simulink subsystem "Controller"  (R2024a)
settings: Solver=VariableStepAuto  StartTime=0.0  StopTime=10.0  RelTol=1e-3
undefined symbols (not defined in the file): A, MPC, N, physics, PWM
libraries: mpclib x3, robotlib x3, simulink x2, ros2lib x2, sharedTrackingLibrary x1
settings Model: Creator=Lamarre  LastModifiedBy=nimai
settings SolverCC: AlgebraicLoopSolver=TrustRegion
settings DebuggingCC: UnconnectedInputMsg=warning  UnconnectedOutputMsg=warning  UnconnectedLineMsg=warning
settings ModelReferenceCC: EnableRefExpFcnMdlSchedulingChecks=on
settings RTWCC: GPUComputeCapability=3.5  DLArmComputeVersion=19.05

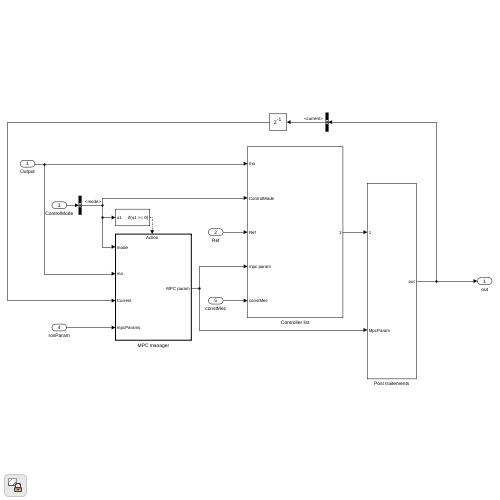
[thumbnail: Simulink's stored preview of the top-level diagram]
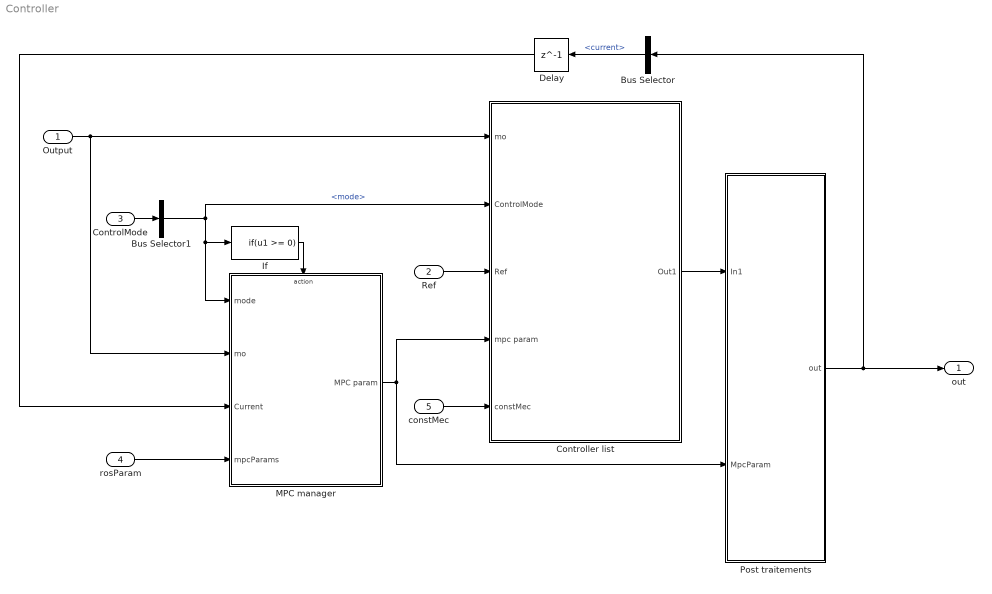
== system Controller ==
  Output : Inport
  Ref : Inport  Port=2
  ControlMode : Inport  Port=3
  rosParam : Inport  Port=4
  constMec : Inport  Port=5
  Bus Selector : BusSelector  OutputSignals=current
  Bus Selector1 : BusSelector  OutputSignals=mode
  Controller list : Subsystem
  Delay : Delay  DelayLength=1  InitialCondition=zeros(1,8)  SampleTime=MPC.Ts
  If : If  IfExpression=u1 >= 0  ShowElse=off
  MPC manager : Subsystem
  Post traitements : Subsystem
  out : Outport
  wires:
  Output/1 -> MPC manager/2(mo), Controller list/1(mo)
  ControlMode/1 -> Bus Selector1/1
  Ref/1 -> Controller list/3(Ref)
  Controller list/1(Out1) -> Post traitements/1(In1)
  Post traitements/1(out) -> out/1, Bus Selector/1
  Delay/1 -> MPC manager/3(Current)
  MPC manager/1(MPC param) -> Post traitements/2(MpcParam), Controller list/4(mpc param)
  Bus Selector/1 -> Delay/1  "<current>"
  Bus Selector1/1 -> Controller list/2(ControlMode), If/1, MPC manager/1(mode)  "<mode>"
  If/1 -> MPC manager/Action
  rosParam/1 -> MPC manager/4(mpcParams)
  constMec/1 -> Controller list/5(constMec)

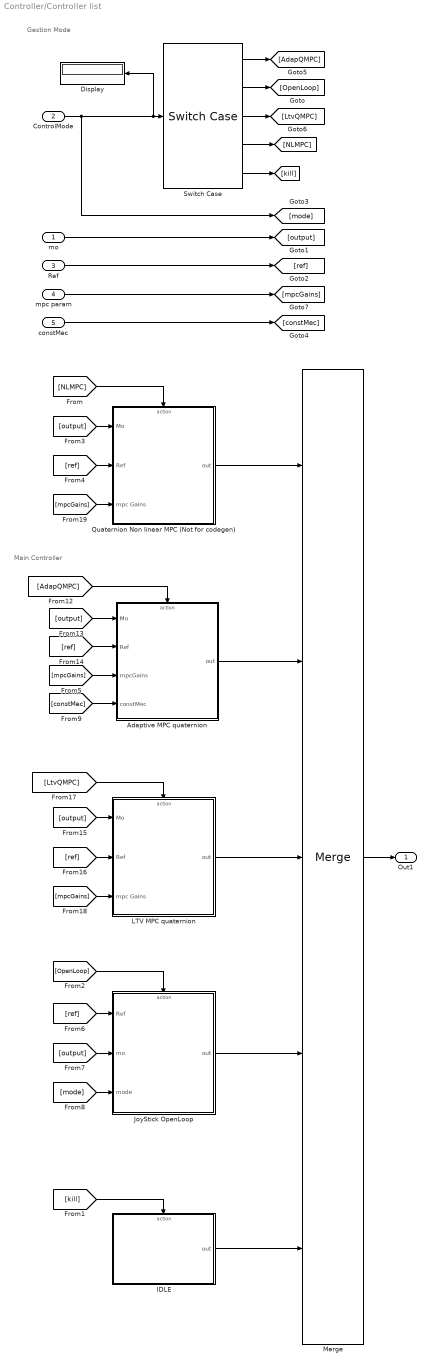
== system Controller/Controller list ==
  note: Gestion Mode
  note: Main Controller
  mo : Inport
  ControlMode : Inport  Port=2
  Ref : Inport  Port=3
  mpc param : Inport  Port=4
  constMec : Inport  Port=5
  "Adaptive MPC quaternion " : Subsystem
  Display : Display
  IDLE : Subsystem  TreatAsAtomicUnit=on
  JoyStick OpenLoop : Subsystem  TreatAsAtomicUnit=on
  "LTV MPC quaternion " : Subsystem
  Merge : Merge  Inputs=5
  Quaternion Non linear MPC (Not for codegen) : Subsystem
  Switch Case : SwitchCase  CaseConditions="{ mode.control.adapQMpcMode,  mode.control.openLoopMode,    mode.control.LtvQMpcMode, mode.control.NlmpcMode}"
  Out1 : Outport
  wires:
  [constMec] -> "Adaptive MPC quaternion "/4(constMec)
  constMec/1 -> [constMec]
  JoyStick OpenLoop/1(out) -> Merge/4
  "LTV MPC quaternion "/1(out) -> Merge/3
  "Adaptive MPC quaternion "/1(out) -> Merge/2
  Switch Case/4 -> [NLMPC]
  Switch Case/3 -> [LtvQMPC]
  Switch Case/1 -> [AdapQMPC]
  [mpcGains] -> Quaternion Non linear MPC (Not for codegen)/3(mpc Gains)
  [mpcGains] -> "LTV MPC quaternion "/3(mpc Gains)
  [mpcGains] -> "Adaptive MPC quaternion "/3(mpcGains)
  mpc param/1 -> [mpcGains]
  Switch Case/2 -> [OpenLoop]
  Ref/1 -> [ref]
  mo/1 -> [output]
  ControlMode/1 -> [mode], Switch Case/1, Display/1
  Switch Case/5 -> [kill]
  [output] -> Quaternion Non linear MPC (Not for codegen)/1(Mo)
  [AdapQMPC] -> "Adaptive MPC quaternion "/Action
  [ref] -> "Adaptive MPC quaternion "/2(Ref)
  [kill] -> IDLE/Action
  [output] -> "LTV MPC quaternion "/1(Mo)
  [ref] -> Quaternion Non linear MPC (Not for codegen)/2(Ref)
  Merge/1 -> Out1/1
  [output] -> JoyStick OpenLoop/2(mo)
  Quaternion Non linear MPC (Not for codegen)/1(out) -> Merge/1
  [ref] -> "LTV MPC quaternion "/2(Ref)
  [output] -> "Adaptive MPC quaternion "/1(Mo)
  [LtvQMPC] -> "LTV MPC quaternion "/Action
  IDLE/1(out) -> Merge/5
  [NLMPC] -> Quaternion Non linear MPC (Not for codegen)/Action
  [mode] -> JoyStick OpenLoop/3(mode)
  [ref] -> JoyStick OpenLoop/1(Ref)
  [OpenLoop] -> JoyStick OpenLoop/Action

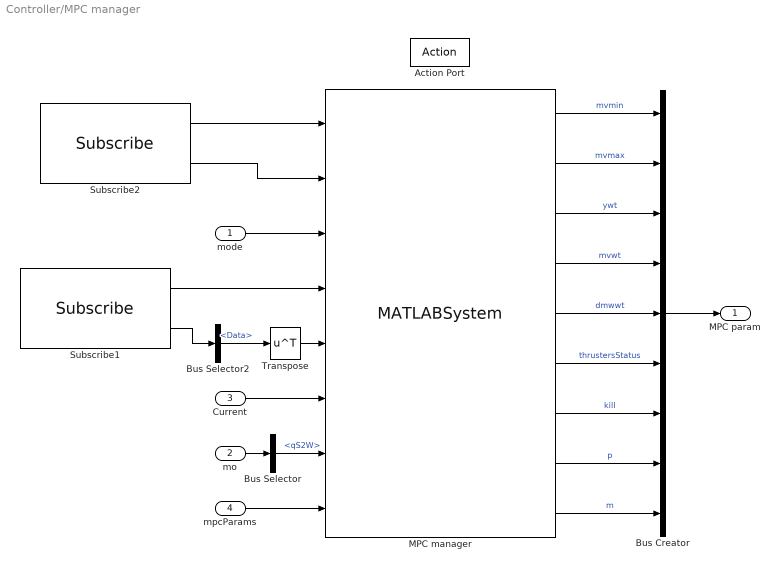
== system Controller/MPC manager ==
  mode : Inport
  mo : Inport  Port=2
  Current : Inport  Port=3
  mpcParams : Inport  Port=4
  Action Port : ActionPort  InitializeStates=reset
  Bus Creator : BusCreator  Inputs=9
  Bus Selector : BusSelector  OutputSignals=qS2W
  Bus Selector2 : BusSelector  OutputSignals=Data
  MPC manager : MATLABSystem  System=mpcManager  mpcConst=MPC  mode=mode  SimulateUsing=Code generation
      mask Type: mpcManager
      mask Display:
      | disp('mpcManager');
      | port_label('input',1,'newRosGains');
      | port_label('input',2,'rosGains');
      | port_label('input',3,'mode');
      | port_label('input',4,'newReadCurrent');
      | port_label('input',5,'readCurrent');
      | port_label('input',6,'estimatedCurrent');
      | port_label('input',7,'mo');
      | port_label('input',8,'mpcParams');
      | port_label('output',1,'mvmin');
      | port_label('output',2,'mvmax');
      | port_label('output',3,'ywt');
      | port_label('output',4,'mvwt');
      | port_label('output',5,'dmwwt');
      | port_label('output',6,'tInfo');
      | port_label('output',7,'kill');
      | port_label('output',8,'p');
      | port_label('output',9,'m');
  Subscribe1 : ros2lib/Subscribe  topicSource=Specify your own  topic=/provider_power/current_not  messageType=std_msgs/Float64MultiArray  sampleTime=-1  QOSHistory=Keep last  QOSDepth=1  QOSReliability=Reliable  QOSDurability=Volatile  QOSDeadline=Inf  QOSLifespan=Inf  QOSLiveliness=Automatic  QOSLeaseDuration=Inf  QOSAvoidROSNamespaceConventions=off
  Subscribe2 : ros2lib/Subscribe  topicSource=Specify your own  topic=/proc_control/set_mpc_gains  messageType=sonia_common_ros2/MpcGains  sampleTime=-1  QOSHistory=Keep last  QOSDepth=1  QOSReliability=Reliable  QOSDurability=Volatile  QOSDeadline=Inf  QOSLifespan=Inf  QOSLiveliness=Automatic  QOSLeaseDuration=Inf  QOSAvoidROSNamespaceConventions=off
  Transpose : Math  Operator=transpose
  MPC param : Outport
  wires:
  mpcParams/1 -> MPC manager/8
  MPC manager/9 -> Bus Creator/9  "m"
  MPC manager/8 -> Bus Creator/8  "p"
  Bus Selector/1 -> MPC manager/7  "<qS2W>"
  mo/1 -> Bus Selector/1
  MPC manager/7 -> Bus Creator/7  "kill"
  MPC manager/6 -> Bus Creator/6  "thrustersStatus"
  Subscribe2/2 -> MPC manager/2
  Subscribe2/1 -> MPC manager/1
  mode/1 -> MPC manager/3
  Subscribe1/1 -> MPC manager/4
  Transpose/1 -> MPC manager/5
  Current/1 -> MPC manager/6
  Bus Creator/1 -> MPC param/1
  MPC manager/3 -> Bus Creator/3  "ywt"
  MPC manager/5 -> Bus Creator/5  "dmwwt"
  MPC manager/4 -> Bus Creator/4  "mvwt"
  MPC manager/2 -> Bus Creator/2  "mvmax"
  MPC manager/1 -> Bus Creator/1  "mvmin"
  Bus Selector2/1 -> Transpose/1  "<Data>"
  Subscribe1/2 -> Bus Selector2/1

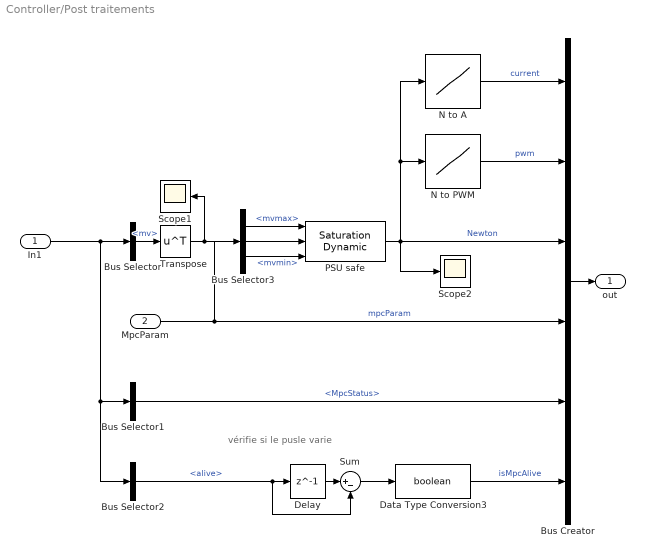
== system Controller/Post traitements ==
  note: vérifie si le pusle varie
  In1 : Inport
  MpcParam : Inport  Port=2
  Bus Creator : BusCreator  Inputs=6
  Bus Selector : BusSelector  OutputSignals=mv
  Bus Selector1 : BusSelector  OutputSignals=MpcStatus
  Bus Selector2 : BusSelector  OutputSignals=alive
  Bus Selector3 : BusSelector  OutputSignals=mvmax,mvmin
  Data Type Conversion3 : DataTypeConversion  OutDataTypeStr=boolean  RndMeth=Nearest  SaturateOnIntegerOverflow=off
  Delay : Delay  DelayLength=1  SampleTime=MPC.Ts
  N to A : Lookup_n-D  NumberOfTableDimensions=1  BreakpointsForDimension1=N  BeginIndexSearchUsingPreviousIndexResult=on  Table=A  InterpMethod=Nearest  ExtrapMethod=Clip  DiagnosticForOutOfRangeInput=Warning  RemoveProtectionInput=on  InternalRulePriority=Speed  OutDataTypeStr=uint16  RndMeth=Simplest
  N to PWM : Lookup_n-D  NumberOfTableDimensions=1  BreakpointsForDimension1=N  BeginIndexSearchUsingPreviousIndexResult=on  Table=PWM  InterpMethod=Nearest  ExtrapMethod=Clip  DiagnosticForOutOfRangeInput=Warning  RemoveProtectionInput=on  InternalRulePriority=Speed  OutDataTypeStr=uint16  RndMeth=Simplest
  PSU safe : simulink/Discontinuities/Saturation Dynamic  OutMin=[]  OutMax=[]  OutDataTypeStr=Inherit: Same as second input  OutDataType=fixdt(1, 16)  OutScaling=2^-10  DoSatur=off
  Scope1 : Scope
  Scope2 : Scope
  Sum : Sum  Inputs=|+-
  Transpose : Math  Operator=transpose
  out : Outport
  wires:
  Bus Selector3/2 -> PSU safe/3  "<mvmin>"
  Bus Selector3/1 -> PSU safe/1  "<mvmax>"
  Transpose/1 -> PSU safe/2, Scope1/1
  Bus Selector2/1 -> Delay/1, Sum/2  "<alive>"
  Data Type Conversion3/1 -> Bus Creator/6  "isMpcAlive"
  Delay/1 -> Sum/1
  Sum/1 -> Data Type Conversion3/1
  MpcParam/1 -> Bus Selector3/1, Bus Creator/4  "mpcParam"
  Bus Creator/1 -> out/1
  N to A/1 -> Bus Creator/1  "current"
  PSU safe/1 -> N to PWM/1, N to A/1, Bus Creator/3, Scope2/1  "Newton"
  In1/1 -> Bus Selector1/1, Bus Selector2/1, Bus Selector/1
  N to PWM/1 -> Bus Creator/2  "pwm"
  Bus Selector/1 -> Transpose/1  "<mv>"
  Bus Selector1/1 -> Bus Creator/5  "<MpcStatus>"

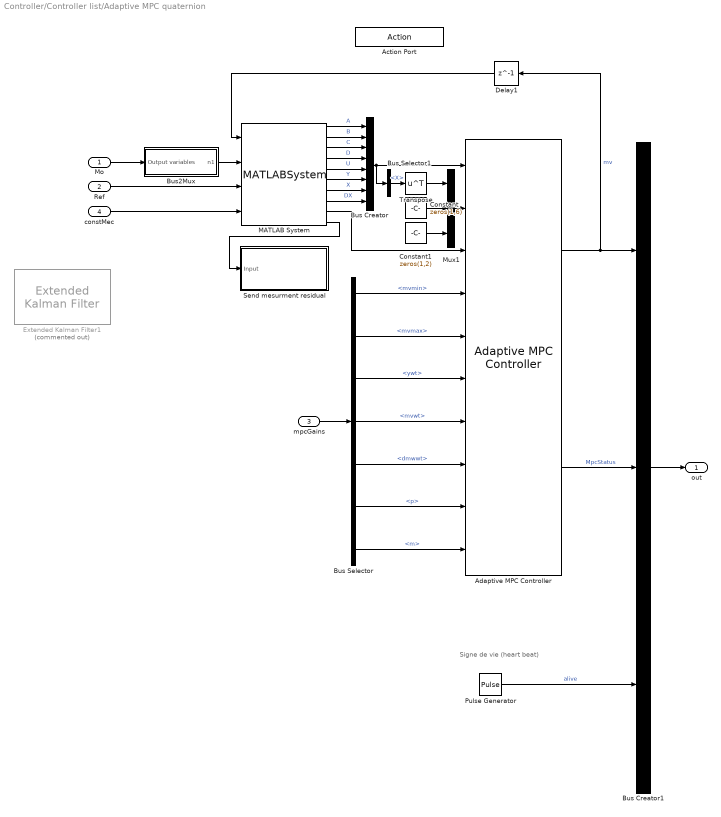
== system Controller/Controller list/Adaptive MPC quaternion  ==
  note: Signe de vie (heart beat)
  Mo : Inport
  Ref : Inport  Port=2
  mpcGains : Inport  Port=3
  constMec : Inport  Port=4
  Action Port : ActionPort  InitializeStates=reset  PropagateVarSize=During execution
  Adaptive MPC Controller : mpclib/Adaptive MPC Controller  SCDEnableBlockLinearizationSpecification=on  mpcobj=Qmpcobj  enable_value=0  updateMPCinCallerWorkspace=on  md_inport=off  mv_inport=off  uref_inport=off  return_cost=off  return_mvseq=off  return_qpstatus=on  return_xseq=off  return_state=off  return_ovseq=off  state_inport=on  isltv_plant=off  umin_inport=on  umax_inport=on  ymin_inport=off  ymax_inport=off  cc_inport=off  ywt_inport=on  uwt_inport=on  duwt_inport=on  rhoeps_inport=off  pm_inport=on  MaximumP=10  HorizonChoice=VariableHorizon  BlockDataType=double  SampleTimeInherited=off  switch_inport=off
  Bus Creator : BusCreator  Inputs=8
  Bus Creator1 : BusCreator  Inputs=3
  Bus Selector : BusSelector  OutputSignals=mvmin,mvmax,ywt,mvwt,dmwwt,p,m
  Bus Selector1 : BusSelector  OutputSignals=X
  Bus2Mux : Subsystem
  Constant : Constant  Value=zeros(1,6)
  Constant1 : Constant  Value=zeros(1,2)
  Delay1 : Delay  DelayLength=1  InitialCondition=zeros(MPC.nu,1)  SampleTime=MPC.Ts
  Extended Kalman Filter1 : sharedTrackingLibrary/Extended Kalman Filter  Commented=on  StateTransitionFcn=QKalmanStateFonction  HasStateTransitionJacobianFcn=off  StateTransitionJacobianFcn=AUVQuatDiscreteJacobianMatrix  HasAdditiveProcessNoise=Additive  ProcessNoise=1  HasTimeVaryingProcessNoise=off  HasStateTransitionFcnExtraArgument=1  InitialState=[0,0,0.31,1,0,0,0,0,0,0,0,0,0,0,0,0,0,0,0,0,0]  InitialStateCovariance=1  MeasurementFcn1=QKalmanMesuredFonction  HasMeasurementJacobianFcn1=off  HasMeasurementEnablePort1=off  HasAdditiveMeasurementNoise1=Additive  MeasurementNoise1=[1,1,1,1,1,1,1,1,1,1,1,1,1]  HasTimeVaryingMeasurementNoise1=off  HasMeasurementFcnExtraArgument1=0  HasMeasurementWrapping1=off  MeasurementFcn2=myMeasurementFcn  HasMeasurementJacobianFcn2=off  HasMeasurementEnablePort2=off  HasAdditiveMeasurementNoise2=Nonadditive  MeasurementNoise2=1  HasTimeVaryingMeasurementNoise2=off  HasMeasurementFcnExtraArgument2=0  HasMeasurementWrapping2=off  MeasurementFcn3=myMeasurementFcn  HasMeasurementJacobianFcn3=off  HasMeasurementEnablePort3=off  HasAdditiveMeasurementNoise3=Additive  MeasurementNoise3=1  HasTimeVaryingMeasurementNoise3=off  HasMeasurementFcnExtraArgument3=0  HasMeasurementWrapping3=off  MeasurementFcn4=myMeasurementFcn  HasMeasurementJacobianFcn4=off  HasMeasurementEnablePort4=off  HasAdditiveMeasurementNoise4=Additive  MeasurementNoise4=1  HasTimeVaryingMeasurementNoise4=off  HasMeasurementFcnExtraArgument4=0  HasMeasurementWrapping4=off  MeasurementFcn5=myMeasurementFcn  HasMeasurementJacobianFcn5=off  HasMeasurementEnablePort5=off  HasAdditiveMeasurementNoise5=Additive  MeasurementNoise5=1  HasTimeVaryingMeasurementNoise5=off  HasMeasurementFcnExtraArgument5=0  HasMeasurementWrapping5=off  EnableMultirate=off  StateTransitionFcnSampleTime=1  MeasurementFcn1SampleTime=1  MeasurementFcn2SampleTime=1  MeasurementFcn3SampleTime=1  MeasurementFcn4SampleTime=1  MeasurementFcn5SampleTime=1  UseCurrentEstimator=on  OutputStateCovariance=off  DataType=double  SampleTime=MPC.Ts  NumberOfMeasurements=1
  MATLAB System : MATLABSystem  System=TrimPlant  MPC=MPC  useDynamicsConst=on  SimulateUsing=Code generation
      mask Type: TrimPlant
      mask Display:
      | disp('TrimPlant');
      | port_label('input',1,'u');
      | port_label('input',2,'y');
      | port_label('input',3,'ref');
      | port_label('input',4,'constMec');
      | port_label('output',1,'A');
      | port_label('output',2,'B');
      | port_label('output',3,'C');
      | port_label('output',4,'D');
      | port_label('output',5,'U');
      | port_label('output',6,'Y');
      | port_label('output',7,'X');
      | port_label('output',8,'DX');
      | port_label('output',9,'ref');
      | port_label('output',10,'Z');
  Mux1 : Mux  Inputs=3
  Pulse Generator : DiscretePulseGenerator  SampleTime=MPC.Ts
  "Send mesurment residual " : Subsystem
  Transpose : Math  Operator=transpose
  out : Outport
  wires:
  MATLAB System/10 -> "Send mesurment residual "/1(Input)
  constMec/1 -> MATLAB System/4
  Bus Selector/7 -> Adaptive MPC Controller/10  "<m>"
  Bus Selector/6 -> Adaptive MPC Controller/9  "<p>"
  Constant1/1 -> Mux1/3
  MATLAB System/9 -> Adaptive MPC Controller/3
  Ref/1 -> MATLAB System/3
  Transpose/1 -> Mux1/1
  Bus Selector1/1 -> Transpose/1  "<X>"
  Mux1/1 -> Adaptive MPC Controller/2
  Bus Selector/5 -> Adaptive MPC Controller/8  "<dmwwt>"
  Bus Selector/4 -> Adaptive MPC Controller/7  "<mvwt>"
  Bus Selector/3 -> Adaptive MPC Controller/6  "<ywt>"
  Bus Selector/2 -> Adaptive MPC Controller/5  "<mvmax>"
  Bus Selector/1 -> Adaptive MPC Controller/4  "<mvmin>"
  mpcGains/1 -> Bus Selector/1
  Constant/1 -> Mux1/2
  Adaptive MPC Controller/1 -> Bus Creator1/1, Delay1/1  "mv"
  Pulse Generator/1 -> Bus Creator1/3  "alive"
  Adaptive MPC Controller/2 -> Bus Creator1/2  "MpcStatus"
  Bus Creator1/1 -> out/1
  Bus2Mux/1(n1) -> MATLAB System/2
  MATLAB System/7 -> Bus Creator/7  "X"
  MATLAB System/6 -> Bus Creator/6  "Y"
  MATLAB System/1 -> Bus Creator/1  "A"
  MATLAB System/8 -> Bus Creator/8  "DX"
  MATLAB System/2 -> Bus Creator/2  "B"
  MATLAB System/5 -> Bus Creator/5  "U"
  Delay1/1 -> MATLAB System/1
  Bus Creator/1 -> Adaptive MPC Controller/1, Bus Selector1/1
  MATLAB System/3 -> Bus Creator/3  "C"
  MATLAB System/4 -> Bus Creator/4  "D"
  Mo/1 -> Bus2Mux/1(Output variables)

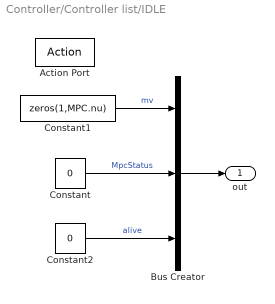
== system Controller/Controller list/IDLE ==
  Action Port : ActionPort
  Bus Creator : BusCreator  Inputs=3
  Constant : Constant  Value=0
  Constant1 : Constant  Value=zeros(1,MPC.nu)
  Constant2 : Constant  Value=0
  out : Outport
  wires:
  Constant1/1 -> Bus Creator/1  "mv"
  Constant2/1 -> Bus Creator/3  "alive"
  Bus Creator/1 -> out/1
  Constant/1 -> Bus Creator/2  "MpcStatus"

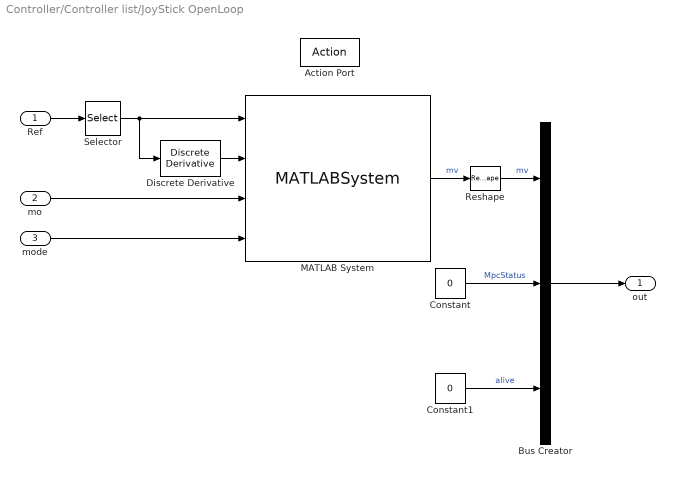
== system Controller/Controller list/JoyStick OpenLoop ==
  Ref : Inport
  mo : Inport  Port=2
  mode : Inport  Port=3
  Action Port : ActionPort
  Bus Creator : BusCreator  Inputs=3
  Constant : Constant  Value=0
  Constant1 : Constant  Value=0
  Discrete Derivative : simulink/Discrete/Discrete Derivative  gainval=1.0  ICPrevScaledInput=0.0  OutMin=[]  OutMax=[]  OutDataType=fixdt(1, 16)  OutScaling=2^-10  DoSatur=off
  MATLAB System : MATLABSystem  System=OpenLoopController  k=40  binv=binv  mass=physics.mass  volume=physics.volume  height=physics.height  I=physics.I  RG=physics.RG  RB=physics.RB  AddedMass=physics.AddedMass  CDL=physics.CDL  CDQ=physics.CDQ  AF=physics.AF  g=physics.g  rho=physics.rho  SimulateUsing=Code generation
      mask Type: OpenLoopController
      mask Display:
      | disp('OpenLoopController');
      | port_label('input',1,'ref');
      | port_label('input',2,'ref_dot');
      | port_label('input',3,'mo');
      | port_label('input',4,'mode');
      | port_label('output',1,'mv');
  Reshape : Reshape
  Selector : Selector  NumberOfDimensions=2  InputPortWidth=13  IndexOptions=Index vector (dialog),Index vector (dialog)  Indices=1,[8:13]  OutputSizes=1,1
  out : Outport
  wires:
  Reshape/1 -> Bus Creator/1  "mv"
  MATLAB System/1 -> Reshape/1  "mv"
  Constant/1 -> Bus Creator/2  "MpcStatus"
  Constant1/1 -> Bus Creator/3  "alive"
  Bus Creator/1 -> out/1
  Selector/1 -> MATLAB System/1, Discrete Derivative/1
  Discrete Derivative/1 -> MATLAB System/2
  Ref/1 -> Selector/1
  mode/1 -> MATLAB System/4
  mo/1 -> MATLAB System/3

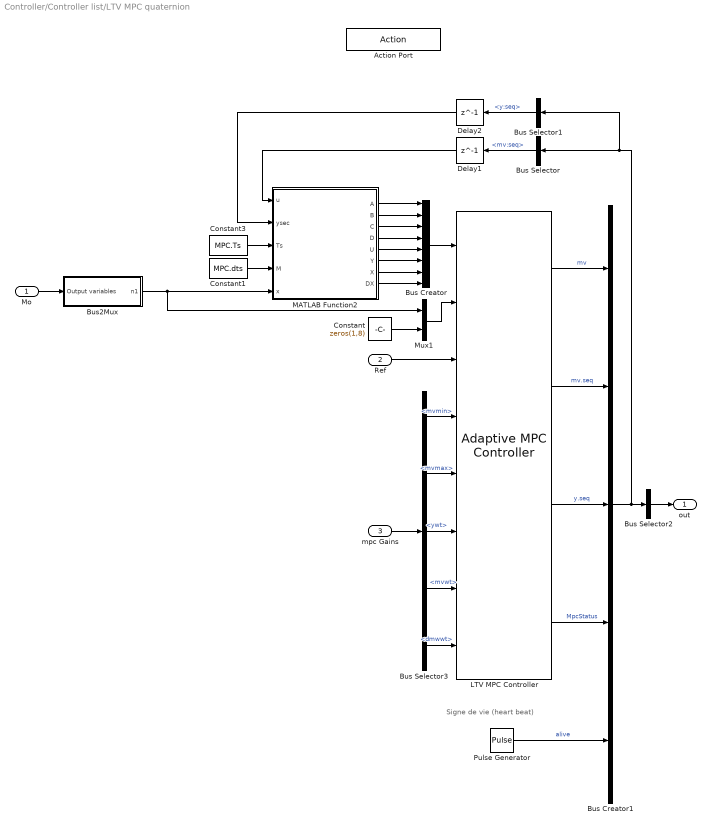
== system Controller/Controller list/LTV MPC quaternion  ==
  note: Signe de vie (heart beat)
  Mo : Inport
  Ref : Inport  Port=2
  mpc Gains : Inport  Port=3
  Action Port : ActionPort  InitializeStates=reset  PropagateVarSize=During execution
  Bus Creator : BusCreator  Inputs=8
  Bus Creator1 : BusCreator  Inputs=5
  Bus Selector : BusSelector  OutputSignals=mv:seq
  Bus Selector1 : BusSelector  OutputSignals=y:seq
  Bus Selector2 : BusSelector  OutputSignals=mv,MpcStatus,alive  OutputAsBus=on
  Bus Selector3 : BusSelector  OutputSignals=mvmin,mvmax,ywt,mvwt,dmwwt
  Bus2Mux : Subsystem
  Constant : Constant  Value=zeros(1,8)
  Constant1 : Constant  Value=MPC.dts
  Constant3 : Constant  Value=MPC.Ts
  Delay1 : Delay  DelayLength=1  InitialCondition=zeros(11,8)  SampleTime=MPC.Ts
  Delay2 : Delay  DelayLength=1  InitialCondition=repmat(MPC.Xi.',11,1)  SampleTime=MPC.Ts
  LTV MPC Controller : mpclib/Adaptive MPC Controller  SCDEnableBlockLinearizationSpecification=on  mpcobj=Qmpcobj  enable_value=0  updateMPCinCallerWorkspace=on  md_inport=off  mv_inport=off  uref_inport=off  return_cost=off  return_mvseq=on  return_qpstatus=on  return_xseq=off  return_state=off  return_ovseq=on  state_inport=on  isltv_plant=on  umin_inport=on  umax_inport=on  ymin_inport=off  ymax_inport=off  cc_inport=off  ywt_inport=on  uwt_inport=on  duwt_inport=on  rhoeps_inport=off  pm_inport=off  MaximumP=10  HorizonChoice=FixedHorizon  BlockDataType=double  SampleTimeInherited=off  switch_inport=off
  MATLAB Function2 : MATLAB Function  TreatAsAtomicUnit=on  SystemSampleTime=MPC.Ts
  Mux1 : Mux  Inputs=2
  Pulse Generator : DiscretePulseGenerator  SampleTime=MPC.Ts
  out : Outport
  wires:
  mpc Gains/1 -> Bus Selector3/1
  Bus Selector3/1 -> LTV MPC Controller/4  "<mvmin>"
  Bus Selector3/2 -> LTV MPC Controller/5  "<mvmax>"
  Bus Selector3/3 -> LTV MPC Controller/6  "<ywt>"
  Bus Selector3/4 -> LTV MPC Controller/7  "<mvwt>"
  Bus Selector3/5 -> LTV MPC Controller/8  "<dmwwt>"
  Bus Selector2/1 -> out/1
  Pulse Generator/1 -> Bus Creator1/5  "alive"
  Bus Selector1/1 -> Delay2/1  "<y:seq>"
  Bus Selector/1 -> Delay1/1  "<mv:seq>"
  Bus Creator1/1 -> Bus Selector2/1, Bus Selector/1, Bus Selector1/1
  LTV MPC Controller/3 -> Bus Creator1/3  "y.seq"
  LTV MPC Controller/4 -> Bus Creator1/4  "MpcStatus"
  LTV MPC Controller/2 -> Bus Creator1/2  "mv.seq"
  LTV MPC Controller/1 -> Bus Creator1/1  "mv"
  Constant/1 -> Mux1/2
  Delay2/1 -> MATLAB Function2/2(ysec)
  Constant1/1 -> MATLAB Function2/4(M)
  Ref/1 -> LTV MPC Controller/3
  Mux1/1 -> LTV MPC Controller/2
  Bus2Mux/1(n1) -> MATLAB Function2/5(x), Mux1/1
  MATLAB Function2/7(X) -> Bus Creator/7
  Constant3/1 -> MATLAB Function2/3(Ts)
  MATLAB Function2/6(Y) -> Bus Creator/6
  MATLAB Function2/1(A) -> Bus Creator/1
  MATLAB Function2/8(DX) -> Bus Creator/8
  MATLAB Function2/2(B) -> Bus Creator/2
  MATLAB Function2/5(U) -> Bus Creator/5
  Delay1/1 -> MATLAB Function2/1(u)
  Bus Creator/1 -> LTV MPC Controller/1
  MATLAB Function2/3(C) -> Bus Creator/3
  MATLAB Function2/4(D) -> Bus Creator/4
  Mo/1 -> Bus2Mux/1(Output variables)

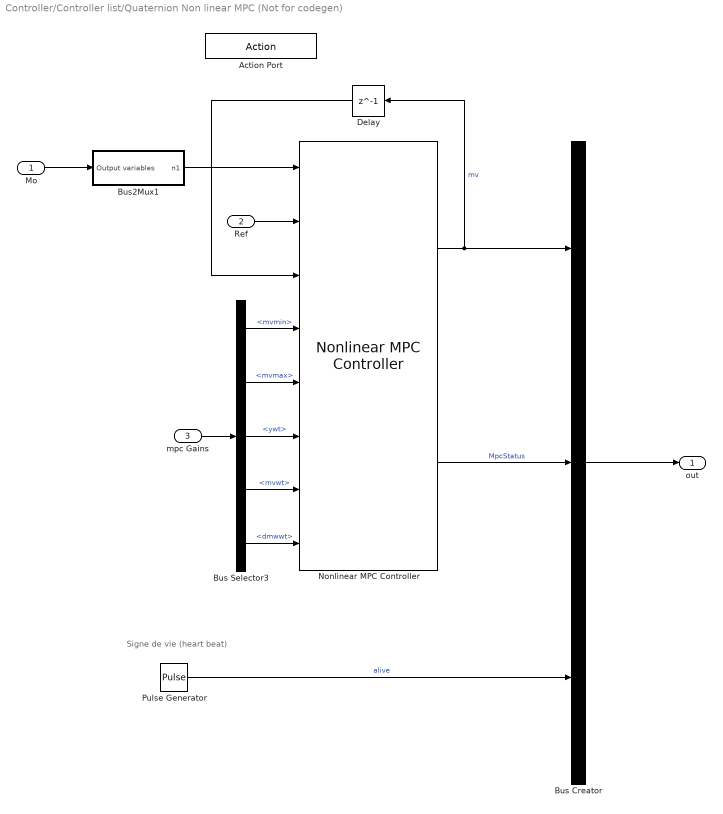
== system Controller/Controller list/Quaternion Non linear MPC (Not for codegen) ==
  note: Signe de vie (heart beat)
  Mo : Inport
  Ref : Inport  Port=2
  mpc Gains : Inport  Port=3
  Action Port : ActionPort  InitializeStates=reset
  Bus Creator : BusCreator  Inputs=3
  Bus Selector3 : BusSelector  OutputSignals=mvmin,mvmax,ywt,mvwt,dmwwt
  Bus2Mux1 : Subsystem
  Delay : Delay  DelayLength=1  InitialCondition=zeros(MPC.nu,1)
  Nonlinear MPC Controller : mpclib/Nonlinear MPC Controller  SCDEnableBlockLinearizationSpecification=on  nlmpcobj=nlobj  UseObjectTs=on  TsControl=mpc.Ts  UseMEX=off  md_enabled=off  mvtarget_enabled=off  param_enabled=off  cost_enabled=off  mvseq_enabled=off  stateseq_enabled=off  ovseq_enabled=off  slack_enabled=off  status_enabled=on  ov_min=off  ov_max=off  mv_min=on  mv_max=on  mvrate_min=off  mvrate_max=off  state_min=off  state_max=off  ov_weight=on  mv_weight=on  mvrate_weight=on  ecr_weight=off  nlp_initialize=off
  Pulse Generator : DiscretePulseGenerator  Period=20  PulseWidth=10  SampleTime=MPC.Ts
  out : Outport
  wires:
  Bus Selector3/1 -> Nonlinear MPC Controller/4  "<mvmin>"
  Bus Selector3/2 -> Nonlinear MPC Controller/5  "<mvmax>"
  mpc Gains/1 -> Bus Selector3/1
  Bus Selector3/4 -> Nonlinear MPC Controller/7  "<mvwt>"
  Bus Selector3/3 -> Nonlinear MPC Controller/6  "<ywt>"
  Bus Selector3/5 -> Nonlinear MPC Controller/8  "<dmwwt>"
  Pulse Generator/1 -> Bus Creator/3  "alive"
  Bus Creator/1 -> out/1
  Nonlinear MPC Controller/2 -> Bus Creator/2  "MpcStatus"
  Delay/1 -> Nonlinear MPC Controller/3
  Ref/1 -> Nonlinear MPC Controller/2
  Nonlinear MPC Controller/1 -> Bus Creator/1, Delay/1  "mv"
  Bus2Mux1/1(n1) -> Nonlinear MPC Controller/1
  Mo/1 -> Bus2Mux1/1(Output variables)

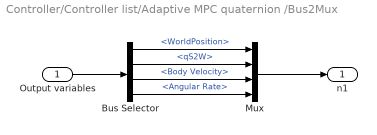
== system Controller/Controller list/Adaptive MPC quaternion /Bus2Mux ==
  Output variables : Inport
  Bus Selector : BusSelector  OutputSignals=WorldPosition,qS2W,Body Velocity,Angular Rate
  Mux : Mux
  n1 : Outport
  wires:
  Bus Selector/2 -> Mux/2  "<qS2W>"
  Bus Selector/3 -> Mux/3  "<Body Velocity>"
  Mux/1 -> n1/1
  Output variables/1 -> Bus Selector/1
  Bus Selector/4 -> Mux/4  "<Angular Rate>"
  Bus Selector/1 -> Mux/1  "<WorldPosition>"

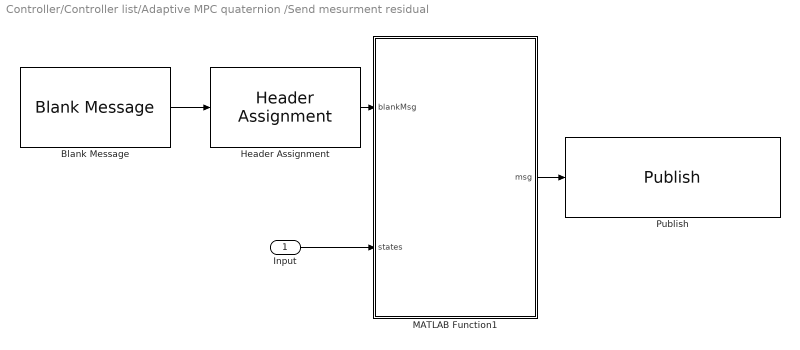
== system Controller/Controller list/Adaptive MPC quaternion /Send mesurment residual  ==
  Input : Inport
  Blank Message : robotlib/Blank Message  messageClass=Message  entityType=nav_msgs/Odometry  messageType=nav_msgs/Odometry  SampleTime=-1  legacyBusStruct=off
  Header Assignment : robotlib/Header Assignment  SetFrameID=on  FrameID=NED  InsertTimeStamp=on  SetHeaderFieldName=Use the default Header field name  HeaderFieldName=Header
  MATLAB Function1 : MATLAB Function  TreatAsAtomicUnit=on
  Publish : robotlib/Publish  topicSource=Specify your own  topic=/proc_control/measurment_residual  messageType=nav_msgs/Odometry  legacyBusStruct=off  messageQueueLength=1
  wires:
  Header Assignment/1 -> MATLAB Function1/1(blankMsg)
  Input/1 -> MATLAB Function1/2(states)
  MATLAB Function1/1(msg) -> Publish/1
  Blank Message/1 -> Header Assignment/1

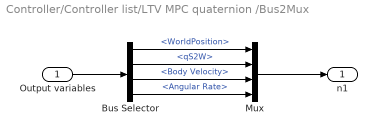
== system Controller/Controller list/LTV MPC quaternion /Bus2Mux ==
  Output variables : Inport
  Bus Selector : BusSelector  OutputSignals=WorldPosition,qS2W,Body Velocity,Angular Rate
  Mux : Mux
  n1 : Outport
  wires:
  Bus Selector/2 -> Mux/2  "<qS2W>"
  Bus Selector/3 -> Mux/3  "<Body Velocity>"
  Mux/1 -> n1/1
  Output variables/1 -> Bus Selector/1
  Bus Selector/4 -> Mux/4  "<Angular Rate>"
  Bus Selector/1 -> Mux/1  "<WorldPosition>"

== system Controller/Controller list/Quaternion Non linear MPC (Not for codegen)/Bus2Mux1 ==
  Output variables : Inport
  Bus Selector : BusSelector  OutputSignals=WorldPosition,qS2W,Body Velocity,Angular Rate
  Mux : Mux
  n1 : Outport
  wires:
  Bus Selector/2 -> Mux/2  "<qS2W>"
  Bus Selector/3 -> Mux/3  "<Body Velocity>"
  Mux/1 -> n1/1
  Output variables/1 -> Bus Selector/1
  Bus Selector/4 -> Mux/4  "<Angular Rate>"
  Bus Selector/1 -> Mux/1  "<WorldPosition>"

== matlab function Controller/Controller list/Adaptive MPC quaternion /Send mesurment residual /MATLAB Function1 ==
  data: blankMsg input; states input; msg output Bus: SL_Bus_proc_control_nav_msgs_Odometry
function msg = SendOdometry(blankMsg, states)
msg = blankMsg;

% World Position 
    msg.Pose.Pose.Position.X = states(1);
    msg.Pose.Pose.Position.Y = states(2);
    msg.Pose.Pose.Position.Z = states(3);
    
% Sub atitude
    msg.Pose.Pose.Orientation.W = states(4);
    msg.Pose.Pose.Orientation.X = states(5);
    msg.Pose.Pose.Orientation.Y = states(6);
    msg.Pose.Pose.Orientation.Z = states(7);

% Body velocity
    msg.Twist.Twist.Linear.X = states(8);
    msg.Twist.Twist.Linear.Y = states(9);
    msg.Twist.Twist.Linear.Z = states(10);
    
% Angular rates
    msg.Twist.Twist.Angular.X = states(11);
    msg.Twist.Twist.Angular.Y = states(12);
    msg.Twist.Twist.Angular.Z = states(13);

== matlab function Controller/Controller list/LTV MPC quaternion /MATLAB Function2 ==
  data: u input; ysec input; Ts input; M input; x input; A output; B output; C output; D output; U output; Y output; X output; DX output
function [A,B,C,D,U,Y,X,DX] = LtvTrimPlantQuat(u,ysec,Ts,M,x)

% Déterminer les dimentions
    nx = size(ysec,2);
    nu = size(u,2);
    p = size(u,1);

% Initialiser les matrices
    A = zeros(nx, nx, p);
    B = zeros(nx, nu, p);
    C = zeros(nx, nx, p);
    D = zeros(nx, nu, p);
    U = zeros(nu, 1, p);
    Y = zeros(13, 1, p);
    X = zeros(13, 1, p);
    DX = zeros(13, 1, p);
    
    
    xkk = x;
for i=1:p
    
    % Actualiser les états
        %xk=ysec(i,:).';
       
            xk=xkk;
      
        
        uk=u(i,:).';
        
    % Lineariser le model dynamique
        [Ac, Bc, C(:,:,i), D(:,:,i)]=AUV8QuatJacobianMatrix(xk,uk);


    % Generate discrete-time model
        A(:,:,i) = expm(Ac*Ts); % Fossen(2021) Eq B.10/B.9 page 662

        BT = Ac(8:13,8:13)\(A(8:13,8:13)-eye(6))*Bc(8:13,1:8); % Fossen(2021) Eq B.11 p 662
        B(:,:,i) = [zeros(7,8); BT];

    % Compute F(x(k+1),u)
       % xkk = ysec()
        % Intégration avec Euler Explicite
        for j=1:M 
          xkk = xkk + AUV8QuatSimFcn(xkk,uk)*(Ts/M);  
          % correct Quaternion
          d=norm(xkk(4:7));
          xkk(4:7) = xkk(4:7)./d;
        end

    % Nominal conditions for discrete-time plant
        U(:,:,i)  = uk.';
        Y(:,:,i)  = xk.';%(Cc*x + Dc*u).';
        X(:,:,i)  = xk.';
        DX(:,:,i) = (xkk-xk).' ;
       
end
disp(X)
end
